simulink model "DC_Step_Resp_Blocks"  (R2013a)
settings: Solver=FixedStepDiscrete  SolverMode=SingleTasking  StartTime=0.0  StopTime=inf  FixedStep=.03  RelTol=1e-3
settings Model: SimulationMode=external  ExtModeTrigDuration=2  Creator=malcoj2  LastModifiedBy=hurstj
settings OptimizationCC: OptimizeModelRefInitCode=on  LifeSpan=1
settings DebuggingCC: SolverPrmCheckMsg=none  StrictBusMsg=Warning
settings HardwareCC: ProdBitPerInt=16  ProdBitPerPointer=8  ProdIntDivRoundTo=Zero  ProdEndianess=LittleEndian  ProdWordSize=8  ProdHWDeviceType=Atmel->AVR
settings RTWCC: SystemTargetFile=realtime.tlc  GenerateMakefile=off  TemplateMakefile=realtime.tmf  Description=Run on Target Hardware  RTWVerbose=off  ProcessScript=realtime_make_rtw_hook
settings STFCustomTargetCC: TargetLibSuffix=.a  GenerateSampleERTMain=on  ERTCustomFileBanners=on  SupportNonInlinedSFcns=off  SupportVariableSizeSignals=on  MATLABClassNameForMDSCustomization=Simulink.SoftwareTarget.ERTCustomization  SystemTargetFile=realtime.tlc
settings ERTTargetCC: ParMdlRefBuildCompliant=off  CompOptLevelCompliant=off  ConcurrentExecutionCompliant=off  CombineOutputUpdateFcns=off  ERTFirstTimeCompliant=off  SupportContinuousTime=on  SupportVariableSizeSignals=on  ModelStepFunctionPrototypeControlCompliant=off  CPPClassGenCompliant=off  ExtMode=on  ExtModeTransport=3  ExtModeMexFile=ext_serial_win32_comm  ExtModeMexArgs=0 1 115200  ERTSrcFileBannerTemplate=realtime_code_template.cgt  ERTHdrFileBannerTemplate=realtime_code_template.cgt  ERTDataSrcFileTemplate=realtime_code_template.cgt  ERTDataHdrFileTemplate=realtime_code_template.cgt  ERTCustomFileTemplate=realtime_file_process.tlc

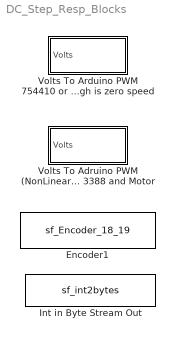
== system DC_Step_Resp_Blocks ==
  Encoder1 : S-Function  InitFcn=try, set_param(gcb,'FunctionName','sf_Encoder_18_19'), end  FunctionName=sf_Encoder_18_19  Parameters=uint8(0),uint8(18),uint8(19)  SFunctionModules=sf_Encoder_18_19_wrapper  EnableBusSupport=off  mask(S-Function Builder){}
      mask init:
      | val = [[.9  0.75 0.75 1 1 .9 .9 1]',[1 1 0.75 0.75 .9 .9 1 .9]'];try , sys = get_param(gcb,'SfunBuilderFcnName');if isempty(sys), sys = get_param(gcb,'FunctionName'); end,catch, sys = get_param(gcb,'FunctionName'); end
      settings: CopyFcn=set_param(gcbh,'LinkStatus','none')  PreSaveFcn=try, set_param(gcb,'FunctionName','sf_Encoder_18_19'), end  OpenFcn=sfunctionwizard(gcbh)
      mask Display: plot(val(:,1),val(:,2)),disp(sys), port_label('output',1,'pos')
  Int in Byte Stream Out : S-Function  InitFcn=try, set_param(gcb,'FunctionName','sf_int2bytes'), end  FunctionName=sf_int2bytes  SFunctionModules=sf_int2bytes_wrapper  EnableBusSupport=off  mask(S-Function Builder){}
      mask init: same as DC_Step_Resp_Blocks/Encoder1
      settings: CopyFcn=set_param(gcb,'LinkStatus','none')  PreSaveFcn=try, set_param(gcb,'FunctionName','sf_int2bytes'), end  OpenFcn=sfunctionwizard(gcbh)
      mask Display: plot(val(:,1),val(:,2)),disp(sys), port_label('input',1,'int_in'), port_label('output',1,'bout')
  Volts To Adruino PWM (NonLinear LOW) 3388 and Motor : Subsystem
  Volts To Arduino PWM 754410 or DRV8833 PWM High is zero speed : Subsystem

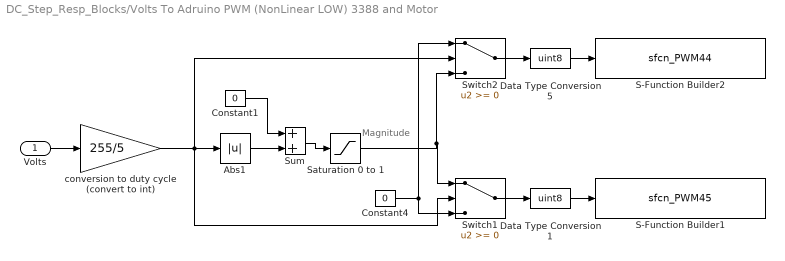
== system DC_Step_Resp_Blocks/Volts To Adruino PWM (NonLinear LOW) 3388 and Motor ==
  note: Magnitude
  Volts : Inport
  Abs1 : Abs
  Constant1 : Constant  Value=0
  Constant4 : Constant  Value=0
  Data Type Conversion1 : DataTypeConversion  OutDataTypeStr=uint8
  Data Type Conversion5 : DataTypeConversion  OutDataTypeStr=uint8
  S-Function Builder1 : S-Function  InitFcn=try, set_param(gcb,'FunctionName','sfcn_PWM45'), end  FunctionName=sfcn_PWM45  Parameters=uint8(45)  SFunctionModules=sfcn_PWM45_wrapper  EnableBusSupport=off  mask(S-Function Builder){}
      mask init: same as DC_Step_Resp_Blocks/Encoder1
      settings: CopyFcn=set_param(gcbh,'LinkStatus','none')  PreSaveFcn=try, set_param(gcb,'FunctionName','sfcn_PWM45'), end  OpenFcn=sfunctionwizard(gcbh)
      mask Display: plot(val(:,1),val(:,2)),disp(sys), port_label('input',1,'in')
  S-Function Builder2 : S-Function  InitFcn=try, set_param(gcb,'FunctionName','sfcn_PWM44'), end  FunctionName=sfcn_PWM44  Parameters=uint8(44)  SFunctionModules=sfcn_PWM44_wrapper  EnableBusSupport=off  mask(S-Function Builder){}
      mask init: same as DC_Step_Resp_Blocks/Encoder1
      settings: CopyFcn=set_param(gcbh,'LinkStatus','none')  PreSaveFcn=try, set_param(gcb,'FunctionName','sfcn_PWM44'), end  OpenFcn=sfunctionwizard(gcbh)
      mask Display: plot(val(:,1),val(:,2)),disp(sys), port_label('input',1,'in')
  Saturation 0 to 1 : Saturate  UpperLimit=255  LowerLimit=0
  Sum : Sum
  Switch1 : Switch
  Switch2 : Switch
  conversion to duty cycle (convert to int) : Gain  Gain=255/5  OutDataTypeStr=int16
  wires:
  Volts/1 -> conversion to duty cycle (convert to int)/1
  conversion to duty cycle (convert to int)/1 -> Switch1/2, Abs1/1, Switch2/2
  Constant4/1 -> Switch2/1, Switch1/3
  Saturation 0 to 1/1 -> Switch2/3, Switch1/1
  Switch2/1 -> Data Type Conversion5/1
  Switch1/1 -> Data Type Conversion1/1
  Data Type Conversion5/1 -> S-Function Builder2/1
  Data Type Conversion1/1 -> S-Function Builder1/1
  Abs1/1 -> Sum/2
  Sum/1 -> Saturation 0 to 1/1
  Constant1/1 -> Sum/1

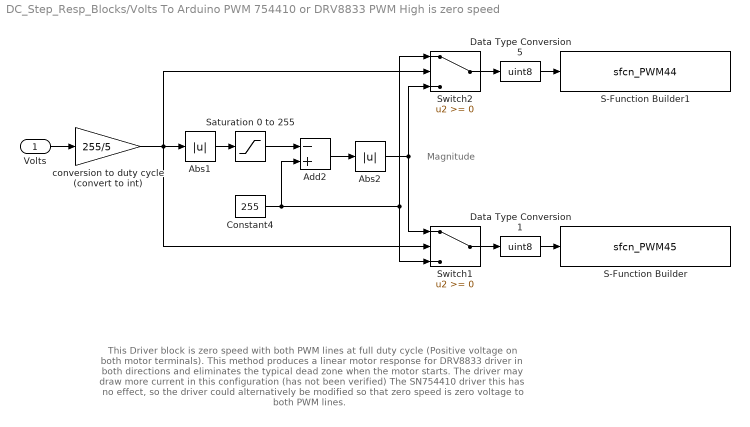
== system DC_Step_Resp_Blocks/Volts To Arduino PWM 754410 or DRV8833 PWM High is zero speed ==
  note: This Driver block is zero speed with both PWM lines at full duty cycle
      |  (Positive voltage on both motor terminals).
      | This method produces a linear motor response for DRV8833 driver
      |  in both directions and eliminates
      | the typical dead zone when the motor starts.
      | The driver may draw more current in this configuration (has not been verified)
      |
      | The SN754410 driver this has no effect, so the driver could alternatively
      | be modified so that zero speed is zero voltage to both PWM lines.
  note: Magnitude
  Volts : Inport
  Abs1 : Abs
  Abs2 : Abs
  Add2 : Sum  Inputs=-+
  Constant4 : Constant  Value=255
  Data Type Conversion1 : DataTypeConversion  OutDataTypeStr=uint8
  Data Type Conversion5 : DataTypeConversion  OutDataTypeStr=uint8
  S-Function Builder : S-Function  InitFcn=try, set_param(gcb,'FunctionName','sfcn_PWM45'), end  FunctionName=sfcn_PWM45  Parameters=uint8(45)  SFunctionModules=sfcn_PWM45_wrapper  EnableBusSupport=off  mask(S-Function Builder){}
      mask init: same as DC_Step_Resp_Blocks/Encoder1
      settings: CopyFcn=set_param(gcbh,'LinkStatus','none')  PreSaveFcn=try, set_param(gcb,'FunctionName','sfcn_PWM45'), end  OpenFcn=sfunctionwizard(gcbh)
      mask Display: plot(val(:,1),val(:,2)),disp(sys), port_label('input',1,'in')
  S-Function Builder1 : S-Function  InitFcn=try, set_param(gcb,'FunctionName','sfcn_PWM44'), end  FunctionName=sfcn_PWM44  Parameters=uint8(44)  SFunctionModules=sfcn_PWM44_wrapper  EnableBusSupport=off  mask(S-Function Builder){}
      mask init: same as DC_Step_Resp_Blocks/Encoder1
      settings: CopyFcn=set_param(gcbh,'LinkStatus','none')  PreSaveFcn=try, set_param(gcb,'FunctionName','sfcn_PWM44'), end  OpenFcn=sfunctionwizard(gcbh)
      mask Display: plot(val(:,1),val(:,2)),disp(sys), port_label('input',1,'in')
  Saturation 0 to 255 : Saturate  UpperLimit=255  LowerLimit=0
  Switch1 : Switch
  Switch2 : Switch
  conversion to duty cycle (convert to int) : Gain  Gain=255/5  OutDataTypeStr=int16
  wires:
  Volts/1 -> conversion to duty cycle (convert to int)/1
  conversion to duty cycle (convert to int)/1 -> Abs1/1, Switch2/2, Switch1/2
  Saturation 0 to 255/1 -> Add2/1
  Abs1/1 -> Saturation 0 to 255/1
  Constant4/1 -> Switch1/3, Switch2/1, Add2/2
  Add2/1 -> Abs2/1
  Abs2/1 -> Switch2/3, Switch1/1
  Switch2/1 -> Data Type Conversion5/1
  Switch1/1 -> Data Type Conversion1/1
  Data Type Conversion5/1 -> S-Function Builder1/1
  Data Type Conversion1/1 -> S-Function Builder/1
